simulink model "ELEC480_1"  (Simulink 7.6)
settings: Solver=ode45  StartTime=0.0  StopTime=10.0  RelTol=1e-3
libraries: simulink x1
settings Model: Creator=ygg001  LastModifiedBy=ygg001

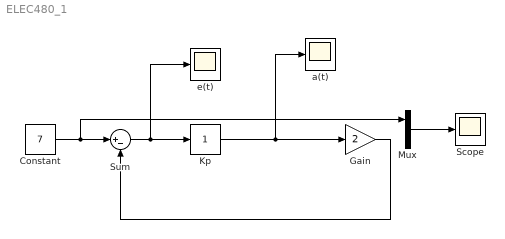
== system ELEC480_1 ==
  Constant : Constant  Value=7
  Gain : Gain  Gain=2
  Kp : simulink/Math Operations/Slider Gain  SystemSampleTime=-1  low=0  gain=1  high=2
  Mux : Mux  Inputs=2
  Scope : Scope
      settings: Tag=c(t) & r
  Sum : Sum  Inputs=|+-
  a(t) : Scope
  e(t) : Scope
      settings: SaveName=ScopeData2
  wires:
  Constant/1 -> Sum/1, Mux/1
  Sum/1 -> Kp/1, e(t)/1
  Kp/1 -> Gain/1, a(t)/1
  Gain/1 -> Sum/2
  Mux/1 -> Scope/1
  ? -> Mux/2
